simulink model "PitchControllerRef"  (R2023b)
settings: Solver=FixedStepDiscrete  StartTime=0.0  StopTime=2  FixedStep=Sample_time  RelTol=1e-3
undefined symbols (not defined in the file): controller_integrator_ic, DiscIntNeverNeededParam, pitch_rate_Ki, pitch_rate_Kp, Sample_time
Description:
  | Referenced 50 Hz pitch-rate PI controller training component.
settings Model: DataDictionary=FCS_Data.sldd  Creator=Tyler  LastModifiedBy=Tyler
settings CodeAppCC: MaxIdLength=63

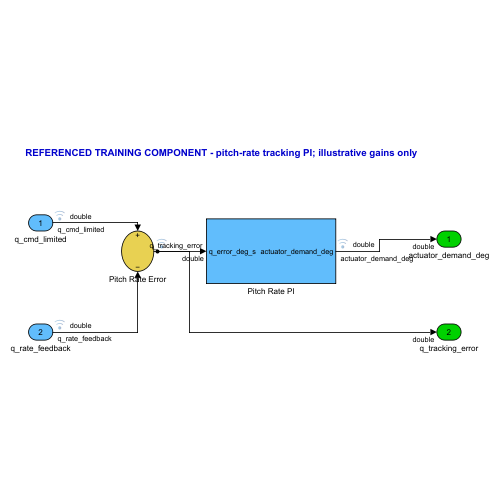
[thumbnail: Simulink's stored preview of the top-level diagram]
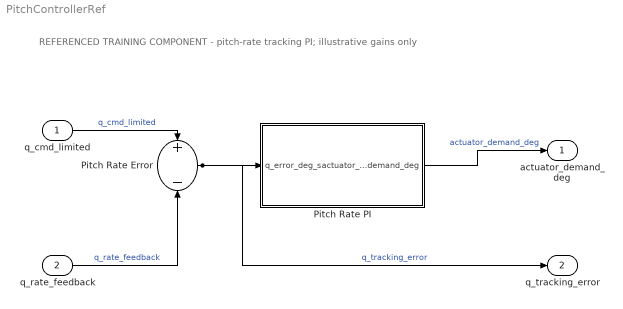
== system PitchControllerRef ==
  note: REFERENCED TRAINING COMPONENT - pitch-rate tracking PI; illustrative gains only
  q_cmd_limited : Inport  OutDataTypeStr=double  Unit=deg/s  SampleTime=Sample_time
  q_rate_feedback : Inport  Port=2  OutDataTypeStr=double  Unit=deg/s  SampleTime=Sample_time
  Pitch Rate Error : Sum  Inputs=+-
  Pitch Rate PI : Subsystem
  actuator_demand_deg : Outport  OutDataTypeStr=double  Unit=deg
  q_tracking_error : Outport  Port=2  OutDataTypeStr=double  Unit=deg/s
  wires:
  q_cmd_limited/1 -> Pitch Rate Error/1  "q_cmd_limited"
  q_rate_feedback/1 -> Pitch Rate Error/2  "q_rate_feedback"
  Pitch Rate Error/1 -> Pitch Rate PI/1(q_error_deg_s), q_tracking_error/1  "q_tracking_error"
  Pitch Rate PI/1(actuator_demand_deg) -> actuator_demand_deg/1  "actuator_demand_deg"

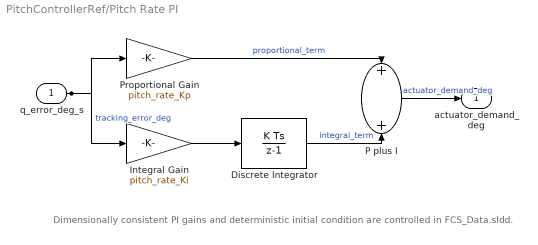
== system PitchControllerRef/Pitch Rate PI ==
  note: Dimensionally consistent PI gains and deterministic initial condition are controlled in FCS_Data.sldd.
  q_error_deg_s : Inport  OutDataTypeStr=double  Unit=deg/s  SampleTime=Sample_time
  Discrete Integrator : DiscreteIntegrator  gainval=1  InitialCondition=controller_integrator_ic  SampleTime=Sample_time  ICPrevOutput=DiscIntNeverNeededParam  ICPrevScaledInput=DiscIntNeverNeededParam
  Integral Gain : Gain  Gain=pitch_rate_Ki
  P plus I : Sum
  Proportional Gain : Gain  Gain=pitch_rate_Kp
  actuator_demand_deg : Outport  OutDataTypeStr=double  Unit=deg
  wires:
  q_error_deg_s/1 -> Proportional Gain/1, Integral Gain/1  "tracking_error_deg"
  Proportional Gain/1 -> P plus I/1  "proportional_term"
  Integral Gain/1 -> Discrete Integrator/1
  Discrete Integrator/1 -> P plus I/2  "integral_term"
  P plus I/1 -> actuator_demand_deg/1  "actuator_demand_deg"
